simulink subsystem "State_Observer"  (R2022b)
settings: Solver=VariableStepAuto  StartTime=0.0  StopTime=10.0  RelTol=1e-3
values from neighbouring files (symbols this model uses):
  Ao = A - L*C    [Observer_Tune.m]
  Bo = [B L]    [Observer_Tune.m]
  Co = eye(3)    [Observer_Tune.m]
  Do = zeros(3, 3)    [Observer_Tune.m]
undefined symbols (not defined in the file or in its folder): bridge
settings Model: Creator=gotta  LastModifiedBy=gotta

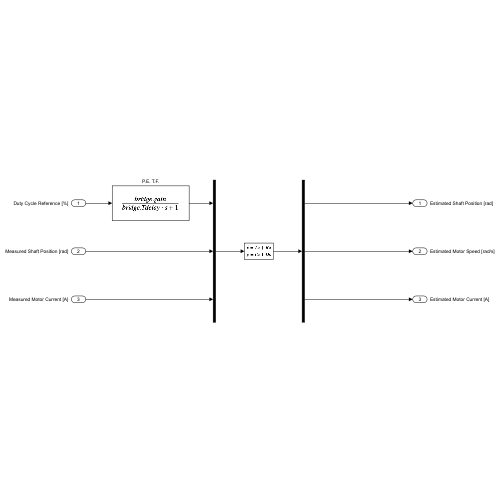
[thumbnail: Simulink's stored preview of the top-level diagram]
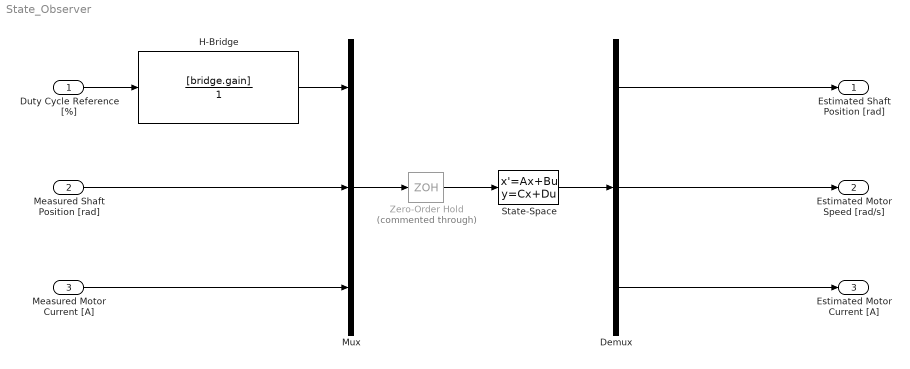
== system State_Observer ==
  Duty Cycle Reference [%] : Inport
  Measured Shaft Position [rad] : Inport  Port=2
  Measured Motor Current [A] : Inport  Port=3
  Demux : Demux  Outputs=3
  H-Bridge : TransferFcn  Numerator=[bridge.gain]  Denominator=[1]
  Mux : Mux  Inputs=3
  State-Space : StateSpace  A=Ao  B=Bo  C=Co  D=Do  InitialCondition=0
  Zero-Order Hold : ZeroOrderHold  Commented=through  SampleTime=-1
  Estimated Shaft Position [rad] : Outport
  Estimated Motor Speed [rad/s] : Outport  Port=2
  Estimated Motor Current [A] : Outport  Port=3
  wires:
  State-Space/1 -> Demux/1
  Mux/1 -> Zero-Order Hold/1
  H-Bridge/1 -> Mux/1
  Demux/1 -> Estimated Shaft Position [rad]/1
  Measured Shaft Position [rad]/1 -> Mux/2
  Duty Cycle Reference [%]/1 -> H-Bridge/1
  Demux/2 -> Estimated Motor Speed [rad/s]/1
  Measured Motor Current [A]/1 -> Mux/3
  Demux/3 -> Estimated Motor Current [A]/1
  Zero-Order Hold/1 -> State-Space/1
